simulink model "ukol7"  (R2024b)
settings: Solver=VariableStepAuto  StartTime=0.0  StopTime=10000  RelTol=1e-3
libraries: slpidlib x6, simulink x2, mpclib x1
settings Model: Creator=jirka  LastModifiedBy=jirka

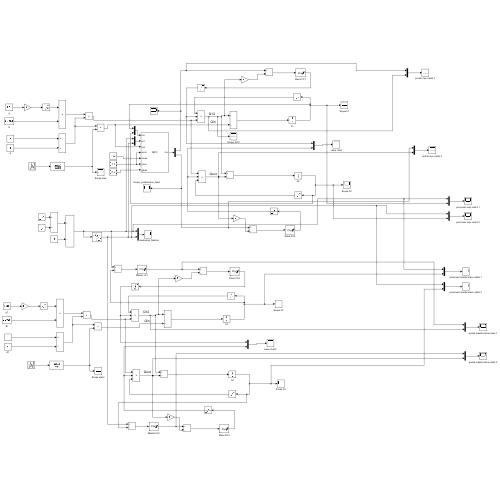
[thumbnail: Simulink's stored preview of the top-level diagram]
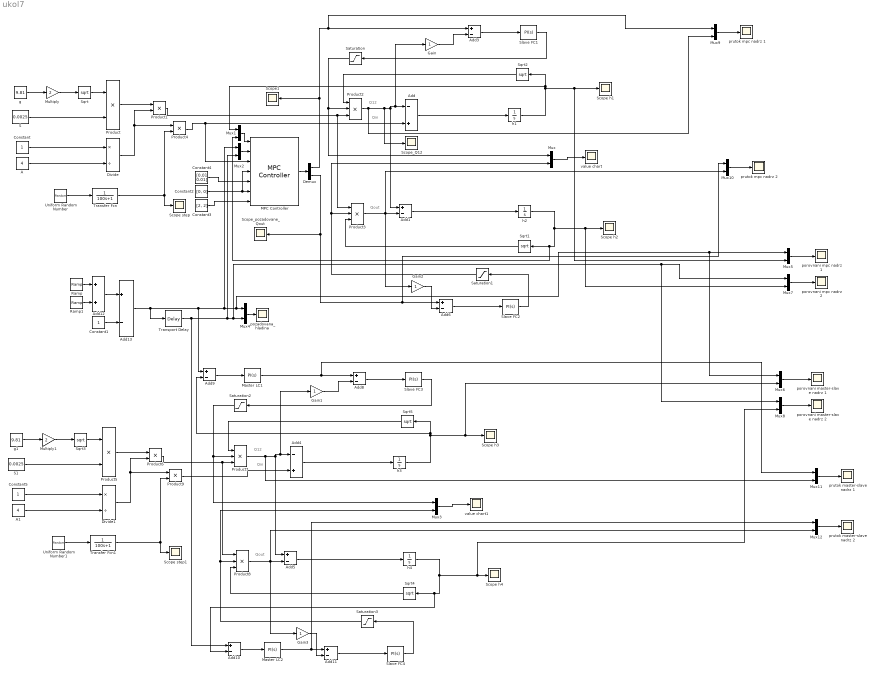
== system ukol7 ==
  note: Qin
  note: Qout
  note: Q12
  note: Qout
  note: Qin
  note: Q12
  A : Constant  Value=4
  A1 : Constant  Value=4
  Add : Sum  Inputs=-+
  Add{1,3,5..6,8..11,13} (9 alike) : Sum  Inputs=+-
  Add12 : Sum
  Add4 : Sum  Inputs=-+
  Constant : Constant
  Constant1 : Constant
  Constant2 : Constant  Value=[0, 0]
  Constant3 : Constant  Value=[2, 2]
  Constant4 : Constant  Value=[0.01 0.01]
  Constant5 : Constant
  Demux : Demux  Outputs=2
  Divide : Product  Inputs=*/
  Divide1 : Product  Inputs=*/
  Gain{,1..3} (4 alike) : Gain
  MPC Controller : mpclib/MPC Controller  SCDEnableBlockLinearizationSpecification=on  mpcobj=mpc1  is_multiple=0  enable_value=0  return_u0=off  updateMPCinCallerWorkspace=on  md_inport=on  mv_inport=off  uref_inport=off  return_cost=off  return_mvseq=off  return_qpstatus=off  return_xseq=off  return_state=off  return_ovseq=off  state_inport=off  umin_inport=on  umax_inport=on  ymin_inport=on  ymax_inport=on  cc_inport=off  ywt_inport=off  uwt_inport=off  duwt_inport=off  rhoeps_inport=off  pm_inport=off  MaximumP=10  HorizonChoice=FixedHorizon  n_ts=0.5  n_p=10  n_mv=2  n_md=1  n_ud=0  n_mo=2  n_uo=0  BlockDataType=double  SampleTimeInherited=off  switch_inport=off
  Master LC1 : slpidlib/PID Controller  Controller=PI  Form=Parallel  TimeDomain=Continuous-time  UseExternalTs=off  SampleTime=-1  IntegratorMethod=Forward Euler  FilterMethod=Forward Euler  ControllerParametersSource=internal  P=-15  I=-1.2  UseKiTs=off  D=0  UseExternalDerivativeSource=off  N=100  UseFilter=on  TunerSelectOption=Transfer Function Based (PID Tuner App)  InitialConditionSource=internal  InitialConditionForIntegrator=0  InitialConditionForFilter=0  DifferentiatorICPrevScaledInput=0  ExternalReset=none  TrackingMode=off  Kt=1  LimitOutput=on  SatLimitsSource=internal  UpperSaturationLimit=inf  LowerSaturationLimit=-inf  LinearizeAsGain=on  AntiWindupMode=back-calculation  Kb=1.2/6  LimitIntegrator=on  UpperIntegratorSaturationLimit=0.01  LowerIntegratorSaturationLimit=0  POutMin=[]  POutMax=[]  IOutMin=[]  IOutMax=[]  DOutMin=[]  DOutMax=[]  NOutMin=[]  NOutMax=[]  SumOutMin=[]  SumOutMax=[]  SaturationOutMin=[]  SaturationOutMax=[]  PParamMin=[]  PParamMax=[]  IParamMin=[]  IParamMax=[]  DParamMin=[]  DParamMax=[]  NParamMin=[]  NParamMax=[]  KbParamMin=[]  KbParamMax=[]  KtParamMin=[]  KtParamMax=[]  KbOutMin=[]  KbOutMax=[]  KtOutMin=[]  KtOutMax=[]  IntegratorOutMin=[]  IntegratorOutMax=[]  FilterOutMin=[]  FilterOutMax=[]  SumI1OutMin=[]  SumI1OutMax=[]  SumI2OutMin=[]  SumI2OutMax=[]  SumI3OutMin=[]  SumI3OutMax=[]  SumI4OutMin=[]  SumI4OutMax=[]  SumDOutMin=[]  SumDOutMax=[]  DifferentiatorOutMin=[]  DifferentiatorOutMax=[]  FilterDiffOutCoefMin=[]  FilterDiffOutCoefMax=[]  ReciprocalOutMin=[]  ReciprocalOutMax=[]  SumDenOutMin=[]  SumDenOutMax=[]  SumNumOutMin=[]  SumNumOutMax=[]  DivideOutMin=[]  DivideOutMax=[]  UdiffTsProdOutMin=[]  UdiffTsProdOutMax=[]  NTsProdOutMin=[]  NTsProdOutMax=[]  UintegralTsProdOutMin=[]  UintegralTsProdOutMax=[]  UngainTsProdOutMin=[]  UngainTsProdOutMax=[]  ClampingZeroOutDataTypeStr=Inherit: Inherit via back propagation  ClampingZeroOutMin=[]  ClampingZeroOutMax=[]  FilterDenConstantOutDataTypeStr=Inherit: Inherit via back propagation  FilterDenConstantOutMin=[]  FilterDenConstantOutMax=[]  PCopyOutDataTypeStr=Inherit: Inherit via back propagation  PCopyOutMin=[]  PCopyOutMax=[]  NCopyOutDataTypeStr=Inherit: Inherit via back propagation  NCopyOutMin=[]  NCopyOutMax=[]  IntegratorContinuousStateAttributes=''  IntegratorStateMustResolveToSignalObject=off  IntegratorRTWStateStorageClass=Auto  FilterContinuousStateAttributes=''  FilterStateMustResolveToSignalObject=off  FilterRTWStateStorageClass=Auto  ParallelPVariant=InternalParameters  IdealPVariant=Disabled  IVariant=InternalParameters  DVariant=Disabled  IntegratorVariant=Continuous  SatVariant=Enabled  AWVariant=BackCalculation  PCopyVariant=Disabled  TRVariant=Disabled  FdbkBlocksVariant=Forward  IdealPFdbkVariant=Disabled  SatFdbkVariant=Disabled  DerivativeFilterVariant=Disabled  NVariant=Disabled  NCopyVariant=Disabled_SignalSpec  FilterICVariant=Disabled  IntegratorICVariant=InternalICs  ExternalResetVariant=Disabled  TRSumVariant=Passthrough  SumFdbkVariant=Disabled  SumVariant=Sum_PI  TsampFilterVariant=InternalTs  TsampNgainVariant=Passthrough  TsampIntegralVariant=Disabled_SignalSpec  ExternalSaturationOutDataTypeStr=Inherit: Same as second input  DerivativeSourceVariant=Disabled  PreIntVariant=InternalPreInt
  Master LC2 : slpidlib/PID Controller  Controller=PI  Form=Parallel  TimeDomain=Continuous-time  UseExternalTs=off  SampleTime=-1  IntegratorMethod=Forward Euler  FilterMethod=Forward Euler  ControllerParametersSource=internal  P=-15  I=-1.2  UseKiTs=off  D=0  UseExternalDerivativeSource=off  N=100  UseFilter=on  TunerSelectOption=Transfer Function Based (PID Tuner App)  InitialConditionSource=internal  InitialConditionForIntegrator=0  InitialConditionForFilter=0  DifferentiatorICPrevScaledInput=0  ExternalReset=none  TrackingMode=off  Kt=1  LimitOutput=on  SatLimitsSource=internal  UpperSaturationLimit=inf  LowerSaturationLimit=-inf  LinearizeAsGain=on  AntiWindupMode=back-calculation  Kb=1.2/6  LimitIntegrator=on  UpperIntegratorSaturationLimit=0.01  LowerIntegratorSaturationLimit=0  POutMin=[]  POutMax=[]  IOutMin=[]  IOutMax=[]  DOutMin=[]  DOutMax=[]  NOutMin=[]  NOutMax=[]  SumOutMin=[]  SumOutMax=[]  SaturationOutMin=[]  SaturationOutMax=[]  PParamMin=[]  PParamMax=[]  IParamMin=[]  IParamMax=[]  DParamMin=[]  DParamMax=[]  NParamMin=[]  NParamMax=[]  KbParamMin=[]  KbParamMax=[]  KtParamMin=[]  KtParamMax=[]  KbOutMin=[]  KbOutMax=[]  KtOutMin=[]  KtOutMax=[]  IntegratorOutMin=[]  IntegratorOutMax=[]  FilterOutMin=[]  FilterOutMax=[]  SumI1OutMin=[]  SumI1OutMax=[]  SumI2OutMin=[]  SumI2OutMax=[]  SumI3OutMin=[]  SumI3OutMax=[]  SumI4OutMin=[]  SumI4OutMax=[]  SumDOutMin=[]  SumDOutMax=[]  DifferentiatorOutMin=[]  DifferentiatorOutMax=[]  FilterDiffOutCoefMin=[]  FilterDiffOutCoefMax=[]  ReciprocalOutMin=[]  ReciprocalOutMax=[]  SumDenOutMin=[]  SumDenOutMax=[]  SumNumOutMin=[]  SumNumOutMax=[]  DivideOutMin=[]  DivideOutMax=[]  UdiffTsProdOutMin=[]  UdiffTsProdOutMax=[]  NTsProdOutMin=[]  NTsProdOutMax=[]  UintegralTsProdOutMin=[]  UintegralTsProdOutMax=[]  UngainTsProdOutMin=[]  UngainTsProdOutMax=[]  ClampingZeroOutDataTypeStr=Inherit: Inherit via back propagation  ClampingZeroOutMin=[]  ClampingZeroOutMax=[]  FilterDenConstantOutDataTypeStr=Inherit: Inherit via back propagation  FilterDenConstantOutMin=[]  FilterDenConstantOutMax=[]  PCopyOutDataTypeStr=Inherit: Inherit via back propagation  PCopyOutMin=[]  PCopyOutMax=[]  NCopyOutDataTypeStr=Inherit: Inherit via back propagation  NCopyOutMin=[]  NCopyOutMax=[]  IntegratorContinuousStateAttributes=''  IntegratorStateMustResolveToSignalObject=off  IntegratorRTWStateStorageClass=Auto  FilterContinuousStateAttributes=''  FilterStateMustResolveToSignalObject=off  FilterRTWStateStorageClass=Auto  ParallelPVariant=InternalParameters  IdealPVariant=Disabled  IVariant=InternalParameters  DVariant=Disabled  IntegratorVariant=Continuous  SatVariant=Enabled  AWVariant=BackCalculation  PCopyVariant=Disabled  TRVariant=Disabled  FdbkBlocksVariant=Forward  IdealPFdbkVariant=Disabled  SatFdbkVariant=Disabled  DerivativeFilterVariant=Disabled  NVariant=Disabled  NCopyVariant=Disabled_SignalSpec  FilterICVariant=Disabled  IntegratorICVariant=InternalICs  ExternalResetVariant=Disabled  TRSumVariant=Passthrough  SumFdbkVariant=Disabled  SumVariant=Sum_PI  TsampFilterVariant=InternalTs  TsampNgainVariant=Passthrough  TsampIntegralVariant=Disabled_SignalSpec  ExternalSaturationOutDataTypeStr=Inherit: Same as second input  DerivativeSourceVariant=Disabled  PreIntVariant=InternalPreInt
  Multiply : Gain  Gain=2
  Multiply1 : Gain  Gain=2
  Mux{,1..12} (13 alike) : Mux  Inputs=2
  Product{,1,4..6,9} (6 alike) : Product
  Product{2..3,7..8} (4 alike) : Product  Inputs=3
  Ramp : simulink/Sources/Ramp  slope=1/5000  start=0  InitialOutput=0
  Ramp1 : simulink/Sources/Ramp  slope=-1/2500  start=5000  InitialOutput=1
  S : Constant  Value=0.0025
  S1 : Constant  Value=0.0025
  Saturation{,1..3} (4 alike) : Saturate  UpperLimit=1  LowerLimit=0
  Scope h{1..4} (4 alike) : Scope
  Scope step : Scope
  Scope step1 : Scope
  Scope1 : Scope
  Scope_Q12 : Scope
  Scope_pozadovane_Qout : Scope
  Slave FC{1..4} (4 alike) : slpidlib/PID Controller  Controller=PI  Form=Parallel  TimeDomain=Continuous-time  UseExternalTs=off  SampleTime=-1  IntegratorMethod=Forward Euler  FilterMethod=Forward Euler  ControllerParametersSource=internal  P=5  I=0.5  UseKiTs=off  D=0  UseExternalDerivativeSource=off  N=100  UseFilter=on  TunerSelectOption=Transfer Function Based (PID Tuner App)  InitialConditionSource=internal  InitialConditionForIntegrator=0  InitialConditionForFilter=0  DifferentiatorICPrevScaledInput=0  ExternalReset=none  TrackingMode=off  Kt=1  LimitOutput=on  SatLimitsSource=internal  UpperSaturationLimit=inf  LowerSaturationLimit=-inf  LinearizeAsGain=on  AntiWindupMode=back-calculation  Kb=0.05/5  LimitIntegrator=on  UpperIntegratorSaturationLimit=1  LowerIntegratorSaturationLimit=0  POutMin=[]  POutMax=[]  IOutMin=[]  IOutMax=[]  DOutMin=[]  DOutMax=[]  NOutMin=[]  NOutMax=[]  SumOutMin=[]  SumOutMax=[]  SaturationOutMin=[]  SaturationOutMax=[]  PParamMin=[]  PParamMax=[]  IParamMin=[]  IParamMax=[]  DParamMin=[]  DParamMax=[]  NParamMin=[]  NParamMax=[]  KbParamMin=[]  KbParamMax=[]  KtParamMin=[]  KtParamMax=[]  KbOutMin=[]  KbOutMax=[]  KtOutMin=[]  KtOutMax=[]  IntegratorOutMin=[]  IntegratorOutMax=[]  FilterOutMin=[]  FilterOutMax=[]  SumI1OutMin=[]  SumI1OutMax=[]  SumI2OutMin=[]  SumI2OutMax=[]  SumI3OutMin=[]  SumI3OutMax=[]  SumI4OutMin=[]  SumI4OutMax=[]  SumDOutMin=[]  SumDOutMax=[]  DifferentiatorOutMin=[]  DifferentiatorOutMax=[]  FilterDiffOutCoefMin=[]  FilterDiffOutCoefMax=[]  ReciprocalOutMin=[]  ReciprocalOutMax=[]  SumDenOutMin=[]  SumDenOutMax=[]  SumNumOutMin=[]  SumNumOutMax=[]  DivideOutMin=[]  DivideOutMax=[]  UdiffTsProdOutMin=[]  UdiffTsProdOutMax=[]  NTsProdOutMin=[]  NTsProdOutMax=[]  UintegralTsProdOutMin=[]  UintegralTsProdOutMax=[]  UngainTsProdOutMin=[]  UngainTsProdOutMax=[]  ClampingZeroOutDataTypeStr=Inherit: Inherit via back propagation  ClampingZeroOutMin=[]  ClampingZeroOutMax=[]  FilterDenConstantOutDataTypeStr=Inherit: Inherit via back propagation  FilterDenConstantOutMin=[]  FilterDenConstantOutMax=[]  PCopyOutDataTypeStr=Inherit: Inherit via back propagation  PCopyOutMin=[]  PCopyOutMax=[]  NCopyOutDataTypeStr=Inherit: Inherit via back propagation  NCopyOutMin=[]  NCopyOutMax=[]  IntegratorContinuousStateAttributes=''  IntegratorStateMustResolveToSignalObject=off  IntegratorRTWStateStorageClass=Auto  FilterContinuousStateAttributes=''  FilterStateMustResolveToSignalObject=off  FilterRTWStateStorageClass=Auto  ParallelPVariant=InternalParameters  IdealPVariant=Disabled  IVariant=InternalParameters  DVariant=Disabled  IntegratorVariant=Continuous  SatVariant=Enabled  AWVariant=BackCalculation  PCopyVariant=Disabled  TRVariant=Disabled  FdbkBlocksVariant=Forward  IdealPFdbkVariant=Disabled  SatFdbkVariant=Disabled  DerivativeFilterVariant=Disabled  NVariant=Disabled  NCopyVariant=Disabled_SignalSpec  FilterICVariant=Disabled  IntegratorICVariant=InternalICs  ExternalResetVariant=Disabled  TRSumVariant=Passthrough  SumFdbkVariant=Disabled  SumVariant=Sum_PI  TsampFilterVariant=InternalTs  TsampNgainVariant=Passthrough  TsampIntegralVariant=Disabled_SignalSpec  ExternalSaturationOutDataTypeStr=Inherit: Same as second input  DerivativeSourceVariant=Disabled  PreIntVariant=InternalPreInt
  Sqrt{,1..5} (6 alike) : Sqrt
  Transfer Fcn : TransferFcn  Denominator=[100 1]
  Transfer Fcn1 : TransferFcn  Denominator=[100 1]
  Transport Delay : TransportDelay  DelayTime=1000
  Uniform Random Number : UniformRandomNumber  Minimum=0.0015  Maximum=0.0085  Seed=984  SampleTime=400
  Uniform Random Number1 : UniformRandomNumber  Minimum=0.0015  Maximum=0.0085  Seed=984  SampleTime=400
  g : Constant  Value=9.81
  g1 : Constant  Value=9.81
  h{1..4} (4 alike) : Integrator  InitialCondition=0.8155
  porovnani master-slave nadrz 1 : Scope
  porovnani master-slave nadrz 2 : Scope
  porovnani mpc nadrz 1 : Scope
  porovnani mpc nadrz 2 : Scope
  pozadovana_hladina : Scope
  prutok master-slave nadrz 1 : Scope
  prutok master-slave nadrz 2 : Scope
  prutok mpc nadrz 1 : Scope
  prutok mpc nadrz 2 : Scope
  value chart : Scope
  value chart1 : Scope
  wires:
  g/1 -> Multiply/1
  Multiply/1 -> Sqrt/1
  Sqrt/1 -> Product/1
  S/1 -> Product/2
  Constant/1 -> Divide/1
  A/1 -> Divide/2
  Product/1 -> Product1/1
  h2/1 -> Mux7/2, Scope h2/1, Mux1/2, Sqrt1/1
  h1/1 -> Mux5/2, Scope h1/1, Sqrt2/1, Mux1/1
  Product2/1 -> Mux9/2, Scope_Q12/1, Gain/1, Add/1, Add1/1
  Sqrt2/1 -> Product2/1
  Product1/1 -> Product3/1, Product2/3
  Sqrt1/1 -> Product3/3
  Product3/1 -> Mux10/2, Add1/2, Gain2/1
  Transfer Fcn/1 -> Product4/2, Scope step/1
  Add/1 -> h1/1
  Add1/1 -> h2/1
  Product4/1 -> MPC Controller/3, Add/2
  Add3/1 -> Slave FC1/1
  Slave FC1/1 -> Saturation/1
  Gain/1 -> Add3/2
  Gain2/1 -> Add6/2
  Slave FC2/1 -> Saturation1/1
  Mux/1 -> value chart/1
  Saturation/1 -> Product2/2, Mux/1
  Saturation1/1 -> Product3/2, Mux/2
  Mux1/1 -> MPC Controller/1
  MPC Controller/1 -> Demux/1
  Demux/2 -> Scope_pozadovane_Qout/1, Mux10/1, Add6/1
  Demux/1 -> Scope1/1, Mux9/1, Add3/1
  Mux2/1 -> MPC Controller/2
  Constant2/1 -> MPC Controller/4, MPC Controller/6
  Constant3/1 -> MPC Controller/7
  Constant4/1 -> MPC Controller/5
  Divide/1 -> Product4/1, Product1/2
  Product9/1 -> Add4/2
  Add8/1 -> Slave FC3/1
  Add10/1 -> Master LC2/1
  Mux3/1 -> value chart1/1
  Add5/1 -> h4/1
  Master LC1/1 -> Mux11/1, Add8/1
  Transfer Fcn1/1 -> Product9/2, Scope step1/1
  Sqrt4/1 -> Product8/3
  Saturation2/1 -> Product7/2, Mux3/1
  Master LC2/1 -> Mux12/1, Add11/1
  Add4/1 -> h3/1
  Add11/1 -> Slave FC4/1
  h3/1 -> Mux6/2, Scope h3/1, Add9/2, Sqrt5/1
  Slave FC3/1 -> Saturation2/1
  g1/1 -> Multiply1/1
  Product5/1 -> Product6/1
  Divide1/1 -> Product9/1, Product6/2
  A1/1 -> Divide1/2
  Gain3/1 -> Add11/2
  S1/1 -> Product5/2
  Product8/1 -> Mux12/2, Add5/2, Gain3/1
  Saturation3/1 -> Mux3/2, Product8/2
  Slave FC4/1 -> Saturation3/1
  Gain1/1 -> Add8/2
  Product7/1 -> Mux11/2, Gain1/1, Add4/1, Add5/1
  Sqrt3/1 -> Product5/1
  Multiply1/1 -> Sqrt3/1
  Add9/1 -> Master LC1/1
  h4/1 -> Mux8/2, Scope h4/1, Add10/2, Sqrt4/1
  Constant5/1 -> Divide1/1
  Product6/1 -> Product8/1, Product7/3
  Sqrt5/1 -> Product7/1
  Ramp/1 -> Add12/1
  Ramp1/1 -> Add12/2
  Add13/1 -> Transport Delay/1, Add9/1, Mux6/1, Mux5/1, Mux4/1, Mux2/1
  Transport Delay/1 -> Mux8/1, Mux7/1, Mux4/2, Mux2/2, Add10/1
  Mux4/1 -> pozadovana_hladina/1
  Add12/1 -> Add13/1
  Constant1/1 -> Add13/2
  Mux6/1 -> porovnani master-slave nadrz 1/1
  Mux5/1 -> porovnani mpc nadrz 1/1
  Mux7/1 -> porovnani mpc nadrz 2/1
  Mux8/1 -> porovnani master-slave nadrz 2/1
  Uniform Random Number/1 -> Transfer Fcn/1
  Uniform Random Number1/1 -> Transfer Fcn1/1
  Mux9/1 -> prutok mpc nadrz 1/1
  Mux10/1 -> prutok mpc nadrz 2/1
  Mux11/1 -> prutok master-slave nadrz 1/1
  Mux12/1 -> prutok master-slave nadrz 2/1
  Add6/1 -> Slave FC2/1
